simulink model "c00002M_harness"  (R2018a)
settings: Solver=FixedStepAuto  StartTime=0.0  StopTime=300  FixedStep=0.1  RelTol=1e-3
undefined symbols (not defined in the file): A1, hmax, R1, R2, sigbuilder_block, TempThreshold
(part 4 of 14)

== system c00002M_harness/M221 ==
  note: VALUES
      | ---------------------------------
      | ControlType = 1 | 2 | 3
      | FillTank = 0 | 1
      | EmptyTank = 0 | 1
      | ManualReference between 0 and 1
      | Tempreature between 0 and 100
      | EmergencyButton = 0 | 1
      | LiquidLevel between 0 and 1 (hmax)
  note: Inputs For Tank2
  note: NAMES
      | --------------------------------------------
      | CT1 = ControlType Tank 1
      | F1 = Fill Tank 1
      | E1 = Empty Tank 1
      | MR1 = Manual Reference Tank1
      | T1 = Temperature Tank 1
      | EB1 = Emergency Button Tank 1
      | LL1 = Liquid Level 1
  note: Inputs For Tank3
  note: Inputs For Tank1
  CT1 : Inport
  MR1 : Inport  Port=2
  T1 : Inport  Port=3
  EB1 : Inport  Port=4
  CT3 : Inport  Port=5
  MR3 : Inport  Port=6
  T3 : Inport  Port=7
  EB3 : Inport  Port=8
  Tank1 : Subsystem
  Tank3 : Subsystem
  LL1 : Outport
  LL3 : Outport  Port=2
  wires:
  EB1/1 -> Tank1/4(EB1)
  Tank3/1(LL3) -> LL3/1
  MR3/1 -> Tank3/2(MR3)
  MR1/1 -> Tank1/2(MR1)
  T1/1 -> Tank1/3(T1)
  Tank1/1(LL1) -> LL1/1
  CT3/1 -> Tank3/1(CT3)
  EB3/1 -> Tank3/4(EB3)
  T3/1 -> Tank3/3(T3)
  CT1/1 -> Tank1/1(CT1)

== system c00002M_harness/M222 ==
  note: VALUES
      | ---------------------------------
      | ControlType = 1 | 2 | 3
      | FillTank = 0 | 1
      | EmptyTank = 0 | 1
      | ManualReference between 0 and 1
      | Tempreature between 0 and 100
      | EmergencyButton = 0 | 1
      | LiquidLevel between 0 and 1 (hmax)
  note: Inputs For Tank2
  note: NAMES
      | --------------------------------------------
      | CT1 = ControlType Tank 1
      | F1 = Fill Tank 1
      | E1 = Empty Tank 1
      | MR1 = Manual Reference Tank1
      | T1 = Temperature Tank 1
      | EB1 = Emergency Button Tank 1
      | LL1 = Liquid Level 1
  note: Inputs For Tank3
  note: Inputs For Tank1
  CT1 : Inport
  MR1 : Inport  Port=2
  T1 : Inport  Port=3
  EB1 : Inport  Port=4
  CT3 : Inport  Port=5
  MR3 : Inport  Port=6
  T3 : Inport  Port=7
  EB3 : Inport  Port=8
  Tank1 : Subsystem
  Tank3 : Subsystem
  LL1 : Outport
  LL3 : Outport  Port=2
  wires:
  EB1/1 -> Tank1/4(EB1)
  Tank3/1(LL3) -> LL3/1
  MR3/1 -> Tank3/2(MR3)
  MR1/1 -> Tank1/2(MR1)
  T1/1 -> Tank1/3(T1)
  Tank1/1(LL1) -> LL1/1
  CT3/1 -> Tank3/1(CT3)
  EB3/1 -> Tank3/4(EB3)
  T3/1 -> Tank3/3(T3)
  CT1/1 -> Tank1/1(CT1)

== system c00002M_harness/M223 ==
  note: VALUES
      | ---------------------------------
      | ControlType = 1 | 2 | 3
      | FillTank = 0 | 1
      | EmptyTank = 0 | 1
      | ManualReference between 0 and 1
      | Tempreature between 0 and 100
      | EmergencyButton = 0 | 1
      | LiquidLevel between 0 and 1 (hmax)
  note: Inputs For Tank2
  note: NAMES
      | --------------------------------------------
      | CT1 = ControlType Tank 1
      | F1 = Fill Tank 1
      | E1 = Empty Tank 1
      | MR1 = Manual Reference Tank1
      | T1 = Temperature Tank 1
      | EB1 = Emergency Button Tank 1
      | LL1 = Liquid Level 1
  note: Inputs For Tank3
  note: Inputs For Tank1
  CT1 : Inport
  MR1 : Inport  Port=2
  T1 : Inport  Port=3
  EB1 : Inport  Port=4
  CT3 : Inport  Port=5
  MR3 : Inport  Port=6
  T3 : Inport  Port=7
  EB3 : Inport  Port=8
  Tank1 : Subsystem
  Tank3 : Subsystem
  LL1 : Outport
  LL3 : Outport  Port=2
  wires:
  EB1/1 -> Tank1/4(EB1)
  Tank3/1(LL3) -> LL3/1
  MR3/1 -> Tank3/2(MR3)
  MR1/1 -> Tank1/2(MR1)
  T1/1 -> Tank1/3(T1)
  Tank1/1(LL1) -> LL1/1
  CT3/1 -> Tank3/1(CT3)
  EB3/1 -> Tank3/4(EB3)
  T3/1 -> Tank3/3(T3)
  CT1/1 -> Tank1/1(CT1)

== system c00002M_harness/M224 ==
  note: VALUES
      | ---------------------------------
      | ControlType = 1 | 2 | 3
      | FillTank = 0 | 1
      | EmptyTank = 0 | 1
      | ManualReference between 0 and 1
      | Tempreature between 0 and 100
      | EmergencyButton = 0 | 1
      | LiquidLevel between 0 and 1 (hmax)
  note: Inputs For Tank2
  note: NAMES
      | --------------------------------------------
      | CT1 = ControlType Tank 1
      | F1 = Fill Tank 1
      | E1 = Empty Tank 1
      | MR1 = Manual Reference Tank1
      | T1 = Temperature Tank 1
      | EB1 = Emergency Button Tank 1
      | LL1 = Liquid Level 1
  note: Inputs For Tank3
  note: Inputs For Tank1
  CT1 : Inport
  MR1 : Inport  Port=2
  T1 : Inport  Port=3
  EB1 : Inport  Port=4
  CT3 : Inport  Port=5
  MR3 : Inport  Port=6
  T3 : Inport  Port=7
  EB3 : Inport  Port=8
  Tank1 : Subsystem
  Tank3 : Subsystem
  LL1 : Outport
  LL3 : Outport  Port=2
  wires:
  EB1/1 -> Tank1/4(EB1)
  Tank3/1(LL3) -> LL3/1
  MR3/1 -> Tank3/2(MR3)
  MR1/1 -> Tank1/2(MR1)
  T1/1 -> Tank1/3(T1)
  Tank1/1(LL1) -> LL1/1
  CT3/1 -> Tank3/1(CT3)
  EB3/1 -> Tank3/4(EB3)
  T3/1 -> Tank3/3(T3)
  CT1/1 -> Tank1/1(CT1)

== system c00002M_harness/M225 ==
  note: VALUES
      | ---------------------------------
      | ControlType = 1 | 2 | 3
      | FillTank = 0 | 1
      | EmptyTank = 0 | 1
      | ManualReference between 0 and 1
      | Tempreature between 0 and 100
      | EmergencyButton = 0 | 1
      | LiquidLevel between 0 and 1 (hmax)
  note: Inputs For Tank2
  note: NAMES
      | --------------------------------------------
      | CT1 = ControlType Tank 1
      | F1 = Fill Tank 1
      | E1 = Empty Tank 1
      | MR1 = Manual Reference Tank1
      | T1 = Temperature Tank 1
      | EB1 = Emergency Button Tank 1
      | LL1 = Liquid Level 1
  note: Inputs For Tank3
  note: Inputs For Tank1
  CT1 : Inport
  MR1 : Inport  Port=2
  T1 : Inport  Port=3
  EB1 : Inport  Port=4
  CT3 : Inport  Port=5
  MR3 : Inport  Port=6
  T3 : Inport  Port=7
  EB3 : Inport  Port=8
  Tank1 : Subsystem
  Tank3 : Subsystem
  LL1 : Outport
  LL3 : Outport  Port=2
  wires:
  EB1/1 -> Tank1/4(EB1)
  Tank3/1(LL3) -> LL3/1
  MR3/1 -> Tank3/2(MR3)
  MR1/1 -> Tank1/2(MR1)
  T1/1 -> Tank1/3(T1)
  Tank1/1(LL1) -> LL1/1
  CT3/1 -> Tank3/1(CT3)
  EB3/1 -> Tank3/4(EB3)
  T3/1 -> Tank3/3(T3)
  CT1/1 -> Tank1/1(CT1)

== system c00002M_harness/M233 ==
  note: VALUES
      | ---------------------------------
      | ControlType = 1 | 2 | 3
      | FillTank = 0 | 1
      | EmptyTank = 0 | 1
      | ManualReference between 0 and 1
      | Tempreature between 0 and 100
      | EmergencyButton = 0 | 1
      | LiquidLevel between 0 and 1 (hmax)
  note: Inputs For Tank2
  note: NAMES
      | --------------------------------------------
      | CT1 = ControlType Tank 1
      | F1 = Fill Tank 1
      | E1 = Empty Tank 1
      | MR1 = Manual Reference Tank1
      | T1 = Temperature Tank 1
      | EB1 = Emergency Button Tank 1
      | LL1 = Liquid Level 1
  note: Inputs For Tank3
  note: Inputs For Tank1
  CT1 : Inport
  MR1 : Inport  Port=2
  T1 : Inport  Port=3
  EB1 : Inport  Port=4
  CT3 : Inport  Port=5
  MR3 : Inport  Port=6
  T3 : Inport  Port=7
  EB3 : Inport  Port=8
  Tank1 : Subsystem
  Tank3 : Subsystem
  LL1 : Outport
  LL3 : Outport  Port=2
  wires:
  EB1/1 -> Tank1/4(EB1)
  Tank3/1(LL3) -> LL3/1
  MR3/1 -> Tank3/2(MR3)
  MR1/1 -> Tank1/2(MR1)
  T1/1 -> Tank1/3(T1)
  Tank1/1(LL1) -> LL1/1
  CT3/1 -> Tank3/1(CT3)
  EB3/1 -> Tank3/4(EB3)
  T3/1 -> Tank3/3(T3)
  CT1/1 -> Tank1/1(CT1)

== system c00002M_harness/M234 ==
  note: VALUES
      | ---------------------------------
      | ControlType = 1 | 2 | 3
      | FillTank = 0 | 1
      | EmptyTank = 0 | 1
      | ManualReference between 0 and 1
      | Tempreature between 0 and 100
      | EmergencyButton = 0 | 1
      | LiquidLevel between 0 and 1 (hmax)
  note: Inputs For Tank2
  note: NAMES
      | --------------------------------------------
      | CT1 = ControlType Tank 1
      | F1 = Fill Tank 1
      | E1 = Empty Tank 1
      | MR1 = Manual Reference Tank1
      | T1 = Temperature Tank 1
      | EB1 = Emergency Button Tank 1
      | LL1 = Liquid Level 1
  note: Inputs For Tank3
  note: Inputs For Tank1
  CT1 : Inport
  MR1 : Inport  Port=2
  T1 : Inport  Port=3
  EB1 : Inport  Port=4
  CT3 : Inport  Port=5
  MR3 : Inport  Port=6
  T3 : Inport  Port=7
  EB3 : Inport  Port=8
  Tank1 : Subsystem
  Tank3 : Subsystem
  LL1 : Outport
  LL3 : Outport  Port=2
  wires:
  EB1/1 -> Tank1/4(EB1)
  Tank3/1(LL3) -> LL3/1
  MR3/1 -> Tank3/2(MR3)
  MR1/1 -> Tank1/2(MR1)
  T1/1 -> Tank1/3(T1)
  Tank1/1(LL1) -> LL1/1
  CT3/1 -> Tank3/1(CT3)
  EB3/1 -> Tank3/4(EB3)
  T3/1 -> Tank3/3(T3)
  CT1/1 -> Tank1/1(CT1)

== system c00002M_harness/M235 ==
  note: VALUES
      | ---------------------------------
      | ControlType = 1 | 2 | 3
      | FillTank = 0 | 1
      | EmptyTank = 0 | 1
      | ManualReference between 0 and 1
      | Tempreature between 0 and 100
      | EmergencyButton = 0 | 1
      | LiquidLevel between 0 and 1 (hmax)
  note: Inputs For Tank2
  note: NAMES
      | --------------------------------------------
      | CT1 = ControlType Tank 1
      | F1 = Fill Tank 1
      | E1 = Empty Tank 1
      | MR1 = Manual Reference Tank1
      | T1 = Temperature Tank 1
      | EB1 = Emergency Button Tank 1
      | LL1 = Liquid Level 1
  note: Inputs For Tank3
  note: Inputs For Tank1
  CT1 : Inport
  MR1 : Inport  Port=2
  T1 : Inport  Port=3
  EB1 : Inport  Port=4
  CT3 : Inport  Port=5
  MR3 : Inport  Port=6
  T3 : Inport  Port=7
  EB3 : Inport  Port=8
  Tank1 : Subsystem
  Tank3 : Subsystem
  LL1 : Outport
  LL3 : Outport  Port=2
  wires:
  EB1/1 -> Tank1/4(EB1)
  Tank3/1(LL3) -> LL3/1
  MR3/1 -> Tank3/2(MR3)
  MR1/1 -> Tank1/2(MR1)
  T1/1 -> Tank1/3(T1)
  Tank1/1(LL1) -> LL1/1
  CT3/1 -> Tank3/1(CT3)
  EB3/1 -> Tank3/4(EB3)
  T3/1 -> Tank3/3(T3)
  CT1/1 -> Tank1/1(CT1)

== system c00002M_harness/M236 ==
  note: VALUES
      | ---------------------------------
      | ControlType = 1 | 2 | 3
      | FillTank = 0 | 1
      | EmptyTank = 0 | 1
      | ManualReference between 0 and 1
      | Tempreature between 0 and 100
      | EmergencyButton = 0 | 1
      | LiquidLevel between 0 and 1 (hmax)
  note: Inputs For Tank2
  note: NAMES
      | --------------------------------------------
      | CT1 = ControlType Tank 1
      | F1 = Fill Tank 1
      | E1 = Empty Tank 1
      | MR1 = Manual Reference Tank1
      | T1 = Temperature Tank 1
      | EB1 = Emergency Button Tank 1
      | LL1 = Liquid Level 1
  note: Inputs For Tank3
  note: Inputs For Tank1
  CT1 : Inport
  MR1 : Inport  Port=2
  T1 : Inport  Port=3
  EB1 : Inport  Port=4
  CT3 : Inport  Port=5
  MR3 : Inport  Port=6
  T3 : Inport  Port=7
  EB3 : Inport  Port=8
  Tank1 : Subsystem
  Tank3 : Subsystem
  LL1 : Outport
  LL3 : Outport  Port=2
  wires:
  EB1/1 -> Tank1/4(EB1)
  Tank3/1(LL3) -> LL3/1
  MR3/1 -> Tank3/2(MR3)
  MR1/1 -> Tank1/2(MR1)
  T1/1 -> Tank1/3(T1)
  Tank1/1(LL1) -> LL1/1
  CT3/1 -> Tank3/1(CT3)
  EB3/1 -> Tank3/4(EB3)
  T3/1 -> Tank3/3(T3)
  CT1/1 -> Tank1/1(CT1)

== system c00002M_harness/M237 ==
  note: VALUES
      | ---------------------------------
      | ControlType = 1 | 2 | 3
      | FillTank = 0 | 1
      | EmptyTank = 0 | 1
      | ManualReference between 0 and 1
      | Tempreature between 0 and 100
      | EmergencyButton = 0 | 1
      | LiquidLevel between 0 and 1 (hmax)
  note: Inputs For Tank2
  note: NAMES
      | --------------------------------------------
      | CT1 = ControlType Tank 1
      | F1 = Fill Tank 1
      | E1 = Empty Tank 1
      | MR1 = Manual Reference Tank1
      | T1 = Temperature Tank 1
      | EB1 = Emergency Button Tank 1
      | LL1 = Liquid Level 1
  note: Inputs For Tank3
  note: Inputs For Tank1
  CT1 : Inport
  MR1 : Inport  Port=2
  T1 : Inport  Port=3
  EB1 : Inport  Port=4
  CT3 : Inport  Port=5
  MR3 : Inport  Port=6
  T3 : Inport  Port=7
  EB3 : Inport  Port=8
  Tank1 : Subsystem
  Tank3 : Subsystem
  LL1 : Outport
  LL3 : Outport  Port=2
  wires:
  EB1/1 -> Tank1/4(EB1)
  Tank3/1(LL3) -> LL3/1
  MR3/1 -> Tank3/2(MR3)
  MR1/1 -> Tank1/2(MR1)
  T1/1 -> Tank1/3(T1)
  Tank1/1(LL1) -> LL1/1
  CT3/1 -> Tank3/1(CT3)
  EB3/1 -> Tank3/4(EB3)
  T3/1 -> Tank3/3(T3)
  CT1/1 -> Tank1/1(CT1)

== system c00002M_harness/M238 ==
  note: VALUES
      | ---------------------------------
      | ControlType = 1 | 2 | 3
      | FillTank = 0 | 1
      | EmptyTank = 0 | 1
      | ManualReference between 0 and 1
      | Tempreature between 0 and 100
      | EmergencyButton = 0 | 1
      | LiquidLevel between 0 and 1 (hmax)
  note: Inputs For Tank2
  note: NAMES
      | --------------------------------------------
      | CT1 = ControlType Tank 1
      | F1 = Fill Tank 1
      | E1 = Empty Tank 1
      | MR1 = Manual Reference Tank1
      | T1 = Temperature Tank 1
      | EB1 = Emergency Button Tank 1
      | LL1 = Liquid Level 1
  note: Inputs For Tank3
  note: Inputs For Tank1
  CT1 : Inport
  MR1 : Inport  Port=2
  T1 : Inport  Port=3
  EB1 : Inport  Port=4
  CT3 : Inport  Port=5
  MR3 : Inport  Port=6
  T3 : Inport  Port=7
  EB3 : Inport  Port=8
  Tank1 : Subsystem
  Tank3 : Subsystem
  LL1 : Outport
  LL3 : Outport  Port=2
  wires:
  EB1/1 -> Tank1/4(EB1)
  Tank3/1(LL3) -> LL3/1
  MR3/1 -> Tank3/2(MR3)
  MR1/1 -> Tank1/2(MR1)
  T1/1 -> Tank1/3(T1)
  Tank1/1(LL1) -> LL1/1
  CT3/1 -> Tank3/1(CT3)
  EB3/1 -> Tank3/4(EB3)
  T3/1 -> Tank3/3(T3)
  CT1/1 -> Tank1/1(CT1)

== system c00002M_harness/M239 ==
  note: VALUES
      | ---------------------------------
      | ControlType = 1 | 2 | 3
      | FillTank = 0 | 1
      | EmptyTank = 0 | 1
      | ManualReference between 0 and 1
      | Tempreature between 0 and 100
      | EmergencyButton = 0 | 1
      | LiquidLevel between 0 and 1 (hmax)
  note: Inputs For Tank2
  note: NAMES
      | --------------------------------------------
      | CT1 = ControlType Tank 1
      | F1 = Fill Tank 1
      | E1 = Empty Tank 1
      | MR1 = Manual Reference Tank1
      | T1 = Temperature Tank 1
      | EB1 = Emergency Button Tank 1
      | LL1 = Liquid Level 1
  note: Inputs For Tank3
  note: Inputs For Tank1
  CT1 : Inport
  MR1 : Inport  Port=2
  T1 : Inport  Port=3
  EB1 : Inport  Port=4
  CT3 : Inport  Port=5
  MR3 : Inport  Port=6
  T3 : Inport  Port=7
  EB3 : Inport  Port=8
  Tank1 : Subsystem
  Tank3 : Subsystem
  LL1 : Outport
  LL3 : Outport  Port=2
  wires:
  EB1/1 -> Tank1/4(EB1)
  Tank3/1(LL3) -> LL3/1
  MR3/1 -> Tank3/2(MR3)
  MR1/1 -> Tank1/2(MR1)
  T1/1 -> Tank1/3(T1)
  Tank1/1(LL1) -> LL1/1
  CT3/1 -> Tank3/1(CT3)
  EB3/1 -> Tank3/4(EB3)
  T3/1 -> Tank3/3(T3)
  CT1/1 -> Tank1/1(CT1)

== system c00002M_harness/M240 ==
  note: VALUES
      | ---------------------------------
      | ControlType = 1 | 2 | 3
      | FillTank = 0 | 1
      | EmptyTank = 0 | 1
      | ManualReference between 0 and 1
      | Tempreature between 0 and 100
      | EmergencyButton = 0 | 1
      | LiquidLevel between 0 and 1 (hmax)
  note: Inputs For Tank2
  note: NAMES
      | --------------------------------------------
      | CT1 = ControlType Tank 1
      | F1 = Fill Tank 1
      | E1 = Empty Tank 1
      | MR1 = Manual Reference Tank1
      | T1 = Temperature Tank 1
      | EB1 = Emergency Button Tank 1
      | LL1 = Liquid Level 1
  note: Inputs For Tank3
  note: Inputs For Tank1
  CT1 : Inport
  MR1 : Inport  Port=2
  T1 : Inport  Port=3
  EB1 : Inport  Port=4
  CT3 : Inport  Port=5
  MR3 : Inport  Port=6
  T3 : Inport  Port=7
  EB3 : Inport  Port=8
  Tank1 : Subsystem
  Tank3 : Subsystem
  LL1 : Outport
  LL3 : Outport  Port=2
  wires:
  EB1/1 -> Tank1/4(EB1)
  Tank3/1(LL3) -> LL3/1
  MR3/1 -> Tank3/2(MR3)
  MR1/1 -> Tank1/2(MR1)
  T1/1 -> Tank1/3(T1)
  Tank1/1(LL1) -> LL1/1
  CT3/1 -> Tank3/1(CT3)
  EB3/1 -> Tank3/4(EB3)
  T3/1 -> Tank3/3(T3)
  CT1/1 -> Tank1/1(CT1)

== system c00002M_harness/M241 ==
  note: VALUES
      | ---------------------------------
      | ControlType = 1 | 2 | 3
      | FillTank = 0 | 1
      | EmptyTank = 0 | 1
      | ManualReference between 0 and 1
      | Tempreature between 0 and 100
      | EmergencyButton = 0 | 1
      | LiquidLevel between 0 and 1 (hmax)
  note: Inputs For Tank2
  note: NAMES
      | --------------------------------------------
      | CT1 = ControlType Tank 1
      | F1 = Fill Tank 1
      | E1 = Empty Tank 1
      | MR1 = Manual Reference Tank1
      | T1 = Temperature Tank 1
      | EB1 = Emergency Button Tank 1
      | LL1 = Liquid Level 1
  note: Inputs For Tank3
  note: Inputs For Tank1
  CT1 : Inport
  MR1 : Inport  Port=2
  T1 : Inport  Port=3
  EB1 : Inport  Port=4
  CT3 : Inport  Port=5
  MR3 : Inport  Port=6
  T3 : Inport  Port=7
  EB3 : Inport  Port=8
  Tank1 : Subsystem
  Tank3 : Subsystem
  LL1 : Outport
  LL3 : Outport  Port=2
  wires:
  EB1/1 -> Tank1/4(EB1)
  Tank3/1(LL3) -> LL3/1
  MR3/1 -> Tank3/2(MR3)
  MR1/1 -> Tank1/2(MR1)
  T1/1 -> Tank1/3(T1)
  Tank1/1(LL1) -> LL1/1
  CT3/1 -> Tank3/1(CT3)
  EB3/1 -> Tank3/4(EB3)
  T3/1 -> Tank3/3(T3)
  CT1/1 -> Tank1/1(CT1)

== system c00002M_harness/M242 ==
  note: VALUES
      | ---------------------------------
      | ControlType = 1 | 2 | 3
      | FillTank = 0 | 1
      | EmptyTank = 0 | 1
      | ManualReference between 0 and 1
      | Tempreature between 0 and 100
      | EmergencyButton = 0 | 1
      | LiquidLevel between 0 and 1 (hmax)
  note: Inputs For Tank2
  note: NAMES
      | --------------------------------------------
      | CT1 = ControlType Tank 1
      | F1 = Fill Tank 1
      | E1 = Empty Tank 1
      | MR1 = Manual Reference Tank1
      | T1 = Temperature Tank 1
      | EB1 = Emergency Button Tank 1
      | LL1 = Liquid Level 1
  note: Inputs For Tank3
  note: Inputs For Tank1
  CT1 : Inport
  MR1 : Inport  Port=2
  T1 : Inport  Port=3
  EB1 : Inport  Port=4
  CT3 : Inport  Port=5
  MR3 : Inport  Port=6
  T3 : Inport  Port=7
  EB3 : Inport  Port=8
  Tank1 : Subsystem
  Tank3 : Subsystem
  LL1 : Outport
  LL3 : Outport  Port=2
  wires:
  EB1/1 -> Tank1/4(EB1)
  Tank3/1(LL3) -> LL3/1
  MR3/1 -> Tank3/2(MR3)
  MR1/1 -> Tank1/2(MR1)
  T1/1 -> Tank1/3(T1)
  Tank1/1(LL1) -> LL1/1
  CT3/1 -> Tank3/1(CT3)
  EB3/1 -> Tank3/4(EB3)
  T3/1 -> Tank3/3(T3)
  CT1/1 -> Tank1/1(CT1)

== system c00002M_harness/M243 ==
  note: VALUES
      | ---------------------------------
      | ControlType = 1 | 2 | 3
      | FillTank = 0 | 1
      | EmptyTank = 0 | 1
      | ManualReference between 0 and 1
      | Tempreature between 0 and 100
      | EmergencyButton = 0 | 1
      | LiquidLevel between 0 and 1 (hmax)
  note: Inputs For Tank2
  note: NAMES
      | --------------------------------------------
      | CT1 = ControlType Tank 1
      | F1 = Fill Tank 1
      | E1 = Empty Tank 1
      | MR1 = Manual Reference Tank1
      | T1 = Temperature Tank 1
      | EB1 = Emergency Button Tank 1
      | LL1 = Liquid Level 1
  note: Inputs For Tank3
  note: Inputs For Tank1
  CT1 : Inport
  MR1 : Inport  Port=2
  T1 : Inport  Port=3
  EB1 : Inport  Port=4
  CT3 : Inport  Port=5
  MR3 : Inport  Port=6
  T3 : Inport  Port=7
  EB3 : Inport  Port=8
  Tank1 : Subsystem
  Tank3 : Subsystem
  LL1 : Outport
  LL3 : Outport  Port=2
  wires:
  EB1/1 -> Tank1/4(EB1)
  Tank3/1(LL3) -> LL3/1
  MR3/1 -> Tank3/2(MR3)
  MR1/1 -> Tank1/2(MR1)
  T1/1 -> Tank1/3(T1)
  Tank1/1(LL1) -> LL1/1
  CT3/1 -> Tank3/1(CT3)
  EB3/1 -> Tank3/4(EB3)
  T3/1 -> Tank3/3(T3)
  CT1/1 -> Tank1/1(CT1)

== system c00002M_harness/M244 ==
  note: VALUES
      | ---------------------------------
      | ControlType = 1 | 2 | 3
      | FillTank = 0 | 1
      | EmptyTank = 0 | 1
      | ManualReference between 0 and 1
      | Tempreature between 0 and 100
      | EmergencyButton = 0 | 1
      | LiquidLevel between 0 and 1 (hmax)
  note: Inputs For Tank2
  note: NAMES
      | --------------------------------------------
      | CT1 = ControlType Tank 1
      | F1 = Fill Tank 1
      | E1 = Empty Tank 1
      | MR1 = Manual Reference Tank1
      | T1 = Temperature Tank 1
      | EB1 = Emergency Button Tank 1
      | LL1 = Liquid Level 1
  note: Inputs For Tank3
  note: Inputs For Tank1
  CT1 : Inport
  MR1 : Inport  Port=2
  T1 : Inport  Port=3
  EB1 : Inport  Port=4
  CT3 : Inport  Port=5
  MR3 : Inport  Port=6
  T3 : Inport  Port=7
  EB3 : Inport  Port=8
  Tank1 : Subsystem
  Tank3 : Subsystem
  LL1 : Outport
  LL3 : Outport  Port=2
  wires:
  EB1/1 -> Tank1/4(EB1)
  Tank3/1(LL3) -> LL3/1
  MR3/1 -> Tank3/2(MR3)
  MR1/1 -> Tank1/2(MR1)
  T1/1 -> Tank1/3(T1)
  Tank1/1(LL1) -> LL1/1
  CT3/1 -> Tank3/1(CT3)
  EB3/1 -> Tank3/4(EB3)
  T3/1 -> Tank3/3(T3)
  CT1/1 -> Tank1/1(CT1)

== system c00002M_harness/M245 ==
  note: VALUES
      | ---------------------------------
      | ControlType = 1 | 2 | 3
      | FillTank = 0 | 1
      | EmptyTank = 0 | 1
      | ManualReference between 0 and 1
      | Tempreature between 0 and 100
      | EmergencyButton = 0 | 1
      | LiquidLevel between 0 and 1 (hmax)
  note: Inputs For Tank2
  note: NAMES
      | --------------------------------------------
      | CT1 = ControlType Tank 1
      | F1 = Fill Tank 1
      | E1 = Empty Tank 1
      | MR1 = Manual Reference Tank1
      | T1 = Temperature Tank 1
      | EB1 = Emergency Button Tank 1
      | LL1 = Liquid Level 1
  note: Inputs For Tank3
  note: Inputs For Tank1
  CT1 : Inport
  MR1 : Inport  Port=2
  T1 : Inport  Port=3
  EB1 : Inport  Port=4
  CT3 : Inport  Port=5
  MR3 : Inport  Port=6
  T3 : Inport  Port=7
  EB3 : Inport  Port=8
  Tank1 : Subsystem
  Tank3 : Subsystem
  LL1 : Outport
  LL3 : Outport  Port=2
  wires:
  EB1/1 -> Tank1/4(EB1)
  Tank3/1(LL3) -> LL3/1
  MR3/1 -> Tank3/2(MR3)
  MR1/1 -> Tank1/2(MR1)
  T1/1 -> Tank1/3(T1)
  Tank1/1(LL1) -> LL1/1
  CT3/1 -> Tank3/1(CT3)
  EB3/1 -> Tank3/4(EB3)
  T3/1 -> Tank3/3(T3)
  CT1/1 -> Tank1/1(CT1)

== system c00002M_harness/M246 ==
  note: VALUES
      | ---------------------------------
      | ControlType = 1 | 2 | 3
      | FillTank = 0 | 1
      | EmptyTank = 0 | 1
      | ManualReference between 0 and 1
      | Tempreature between 0 and 100
      | EmergencyButton = 0 | 1
      | LiquidLevel between 0 and 1 (hmax)
  note: Inputs For Tank2
  note: NAMES
      | --------------------------------------------
      | CT1 = ControlType Tank 1
      | F1 = Fill Tank 1
      | E1 = Empty Tank 1
      | MR1 = Manual Reference Tank1
      | T1 = Temperature Tank 1
      | EB1 = Emergency Button Tank 1
      | LL1 = Liquid Level 1
  note: Inputs For Tank3
  note: Inputs For Tank1
  CT1 : Inport
  MR1 : Inport  Port=2
  T1 : Inport  Port=3
  EB1 : Inport  Port=4
  CT3 : Inport  Port=5
  MR3 : Inport  Port=6
  T3 : Inport  Port=7
  EB3 : Inport  Port=8
  Tank1 : Subsystem
  Tank3 : Subsystem
  LL1 : Outport
  LL3 : Outport  Port=2
  wires:
  EB1/1 -> Tank1/4(EB1)
  Tank3/1(LL3) -> LL3/1
  MR3/1 -> Tank3/2(MR3)
  MR1/1 -> Tank1/2(MR1)
  T1/1 -> Tank1/3(T1)
  Tank1/1(LL1) -> LL1/1
  CT3/1 -> Tank3/1(CT3)
  EB3/1 -> Tank3/4(EB3)
  T3/1 -> Tank3/3(T3)
  CT1/1 -> Tank1/1(CT1)

== system c00002M_harness/CPSUT/Tank1 ==
  CT1 : Inport
  MR1 : Inport  Port=2
  T1 : Inport  Port=3
  EB1 : Inport  Port=4
  Control : Subsystem
  Memory : Memory
  TankModel : Subsystem
  LL1 : Outport
  wires:
  TankModel/1(LiquidLevel) -> Memory/1, LL1/1
  Control/2(LiquidOut) -> TankModel/2(LiquidOut)
  Memory/1 -> Control/5(LiquidLevel)
  MR1/1 -> Control/2(ManualReference)
  CT1/1 -> Control/1(ControlType)
  EB1/1 -> Control/3(EmergencyButton)
  T1/1 -> Control/4(Temperature)
  Control/1(LiquidIn) -> TankModel/1(LiquidIn)

== system c00002M_harness/CPSUT/Tank3 ==
  CT3 : Inport
  MR3 : Inport  Port=2
  T3 : Inport  Port=3
  EB3 : Inport  Port=4
  Control : Subsystem
  Memory : Memory
  TankModel : Subsystem
  LL3 : Outport
  wires:
  TankModel/1(LiquidLevel) -> Memory/1, LL3/1
  Control/2(LiquidOut) -> TankModel/2(LiquidOut)
  Memory/1 -> Control/5(LiquidLevel)
  MR3/1 -> Control/2(ManualReference)
  CT3/1 -> Control/1(ControlType)
  EB3/1 -> Control/3(EmergencyButton)
  T3/1 -> Control/4(Temperature)
  Control/1(LiquidIn) -> TankModel/1(LiquidIn)

== system c00002M_harness/M001/Tank1 ==
  CT1 : Inport
  MR1 : Inport  Port=2
  T1 : Inport  Port=3
  EB1 : Inport  Port=4
  Control : Subsystem
  Memory : Memory
  TankModel : Subsystem
  LL1 : Outport
  wires:
  T1/1 -> Control/4(Temperature)
  EB1/1 -> Control/3(EmergencyButton)
  CT1/1 -> Control/1(ControlType)
  MR1/1 -> Control/2(ManualReference)
  Memory/1 -> Control/5(LiquidLevel)
  Control/2(LiquidOut) -> TankModel/2(LiquidOut)
  TankModel/1(LiquidLevel) -> LL1/1, Memory/1
  Control/1(LiquidIn) -> TankModel/1(LiquidIn)

== system c00002M_harness/M001/Tank3 ==
  CT3 : Inport
  MR3 : Inport  Port=2
  T3 : Inport  Port=3
  EB3 : Inport  Port=4
  Control : Subsystem
  Memory : Memory
  TankModel : Subsystem
  LL3 : Outport
  wires:
  T3/1 -> Control/4(Temperature)
  EB3/1 -> Control/3(EmergencyButton)
  CT3/1 -> Control/1(ControlType)
  MR3/1 -> Control/2(ManualReference)
  Memory/1 -> Control/5(LiquidLevel)
  Control/2(LiquidOut) -> TankModel/2(LiquidOut)
  TankModel/1(LiquidLevel) -> LL3/1, Memory/1
  Control/1(LiquidIn) -> TankModel/1(LiquidIn)

== system c00002M_harness/M002/Tank1 ==
  CT1 : Inport
  MR1 : Inport  Port=2
  T1 : Inport  Port=3
  EB1 : Inport  Port=4
  Control : Subsystem
  Memory : Memory
  TankModel : Subsystem
  LL1 : Outport
  wires:
  TankModel/1(LiquidLevel) -> Memory/1, LL1/1
  Control/2(LiquidOut) -> TankModel/2(LiquidOut)
  Memory/1 -> Control/5(LiquidLevel)
  MR1/1 -> Control/2(ManualReference)
  CT1/1 -> Control/1(ControlType)
  EB1/1 -> Control/3(EmergencyButton)
  T1/1 -> Control/4(Temperature)
  Control/1(LiquidIn) -> TankModel/1(LiquidIn)

== system c00002M_harness/M002/Tank3 ==
  CT3 : Inport
  MR3 : Inport  Port=2
  T3 : Inport  Port=3
  EB3 : Inport  Port=4
  Control : Subsystem
  Memory : Memory
  TankModel : Subsystem
  LL3 : Outport
  wires:
  TankModel/1(LiquidLevel) -> Memory/1, LL3/1
  Control/2(LiquidOut) -> TankModel/2(LiquidOut)
  Memory/1 -> Control/5(LiquidLevel)
  MR3/1 -> Control/2(ManualReference)
  CT3/1 -> Control/1(ControlType)
  EB3/1 -> Control/3(EmergencyButton)
  T3/1 -> Control/4(Temperature)
  Control/1(LiquidIn) -> TankModel/1(LiquidIn)

== system c00002M_harness/M003/Tank1 ==
  CT1 : Inport
  MR1 : Inport  Port=2
  T1 : Inport  Port=3
  EB1 : Inport  Port=4
  Control : Subsystem
  Memory : Memory
  TankModel : Subsystem
  LL1 : Outport
  wires:
  TankModel/1(LiquidLevel) -> Memory/1, LL1/1
  Control/2(LiquidOut) -> TankModel/2(LiquidOut)
  Memory/1 -> Control/5(LiquidLevel)
  MR1/1 -> Control/2(ManualReference)
  CT1/1 -> Control/1(ControlType)
  EB1/1 -> Control/3(EmergencyButton)
  T1/1 -> Control/4(Temperature)
  Control/1(LiquidIn) -> TankModel/1(LiquidIn)

== system c00002M_harness/M003/Tank3 ==
  CT3 : Inport
  MR3 : Inport  Port=2
  T3 : Inport  Port=3
  EB3 : Inport  Port=4
  Control : Subsystem
  Memory : Memory
  TankModel : Subsystem
  LL3 : Outport
  wires:
  TankModel/1(LiquidLevel) -> Memory/1, LL3/1
  Control/2(LiquidOut) -> TankModel/2(LiquidOut)
  Memory/1 -> Control/5(LiquidLevel)
  MR3/1 -> Control/2(ManualReference)
  CT3/1 -> Control/1(ControlType)
  EB3/1 -> Control/3(EmergencyButton)
  T3/1 -> Control/4(Temperature)
  Control/1(LiquidIn) -> TankModel/1(LiquidIn)

== system c00002M_harness/M004/Tank1 ==
  CT1 : Inport
  MR1 : Inport  Port=2
  T1 : Inport  Port=3
  EB1 : Inport  Port=4
  Control : Subsystem
  Memory : Memory
  TankModel : Subsystem
  LL1 : Outport
  wires:
  TankModel/1(LiquidLevel) -> Memory/1, LL1/1
  Control/2(LiquidOut) -> TankModel/2(LiquidOut)
  Memory/1 -> Control/5(LiquidLevel)
  MR1/1 -> Control/2(ManualReference)
  CT1/1 -> Control/1(ControlType)
  EB1/1 -> Control/3(EmergencyButton)
  T1/1 -> Control/4(Temperature)
  Control/1(LiquidIn) -> TankModel/1(LiquidIn)

== system c00002M_harness/M004/Tank3 ==
  CT3 : Inport
  MR3 : Inport  Port=2
  T3 : Inport  Port=3
  EB3 : Inport  Port=4
  Control : Subsystem
  Memory : Memory
  TankModel : Subsystem
  LL3 : Outport
  wires:
  TankModel/1(LiquidLevel) -> Memory/1, LL3/1
  Control/2(LiquidOut) -> TankModel/2(LiquidOut)
  Memory/1 -> Control/5(LiquidLevel)
  MR3/1 -> Control/2(ManualReference)
  CT3/1 -> Control/1(ControlType)
  EB3/1 -> Control/3(EmergencyButton)
  T3/1 -> Control/4(Temperature)
  Control/1(LiquidIn) -> TankModel/1(LiquidIn)

== system c00002M_harness/M046/Tank1 ==
  CT1 : Inport
  MR1 : Inport  Port=2
  T1 : Inport  Port=3
  EB1 : Inport  Port=4
  Control : Subsystem
  Memory : Memory
  TankModel : Subsystem
  LL1 : Outport
  wires:
  TankModel/1(LiquidLevel) -> Memory/1, LL1/1
  Control/2(LiquidOut) -> TankModel/2(LiquidOut)
  Memory/1 -> Control/5(LiquidLevel)
  MR1/1 -> Control/2(ManualReference)
  CT1/1 -> Control/1(ControlType)
  EB1/1 -> Control/3(EmergencyButton)
  T1/1 -> Control/4(Temperature)
  Control/1(LiquidIn) -> TankModel/1(LiquidIn)

== system c00002M_harness/M046/Tank3 ==
  CT3 : Inport
  MR3 : Inport  Port=2
  T3 : Inport  Port=3
  EB3 : Inport  Port=4
  Control : Subsystem
  Memory : Memory
  TankModel : Subsystem
  LL3 : Outport
  wires:
  TankModel/1(LiquidLevel) -> Memory/1, LL3/1
  Control/2(LiquidOut) -> TankModel/2(LiquidOut)
  Memory/1 -> Control/5(LiquidLevel)
  MR3/1 -> Control/2(ManualReference)
  CT3/1 -> Control/1(ControlType)
  EB3/1 -> Control/3(EmergencyButton)
  T3/1 -> Control/4(Temperature)
  Control/1(LiquidIn) -> TankModel/1(LiquidIn)

== system c00002M_harness/M047/Tank1 ==
  CT1 : Inport
  MR1 : Inport  Port=2
  T1 : Inport  Port=3
  EB1 : Inport  Port=4
  Control : Subsystem
  Memory : Memory
  TankModel : Subsystem
  LL1 : Outport
  wires:
  TankModel/1(LiquidLevel) -> Memory/1, LL1/1
  Control/2(LiquidOut) -> TankModel/2(LiquidOut)
  Memory/1 -> Control/5(LiquidLevel)
  MR1/1 -> Control/2(ManualReference)
  CT1/1 -> Control/1(ControlType)
  EB1/1 -> Control/3(EmergencyButton)
  T1/1 -> Control/4(Temperature)
  Control/1(LiquidIn) -> TankModel/1(LiquidIn)

== system c00002M_harness/M047/Tank3 ==
  CT3 : Inport
  MR3 : Inport  Port=2
  T3 : Inport  Port=3
  EB3 : Inport  Port=4
  Control : Subsystem
  Memory : Memory
  TankModel : Subsystem
  LL3 : Outport
  wires:
  TankModel/1(LiquidLevel) -> Memory/1, LL3/1
  Control/2(LiquidOut) -> TankModel/2(LiquidOut)
  Memory/1 -> Control/5(LiquidLevel)
  MR3/1 -> Control/2(ManualReference)
  CT3/1 -> Control/1(ControlType)
  EB3/1 -> Control/3(EmergencyButton)
  T3/1 -> Control/4(Temperature)
  Control/1(LiquidIn) -> TankModel/1(LiquidIn)

== system c00002M_harness/M048/Tank1 ==
  CT1 : Inport
  MR1 : Inport  Port=2
  T1 : Inport  Port=3
  EB1 : Inport  Port=4
  Control : Subsystem
  Memory : Memory
  TankModel : Subsystem
  LL1 : Outport
  wires:
  TankModel/1(LiquidLevel) -> Memory/1, LL1/1
  Control/2(LiquidOut) -> TankModel/2(LiquidOut)
  Memory/1 -> Control/5(LiquidLevel)
  MR1/1 -> Control/2(ManualReference)
  CT1/1 -> Control/1(ControlType)
  EB1/1 -> Control/3(EmergencyButton)
  T1/1 -> Control/4(Temperature)
  Control/1(LiquidIn) -> TankModel/1(LiquidIn)

== system c00002M_harness/M048/Tank3 ==
  CT3 : Inport
  MR3 : Inport  Port=2
  T3 : Inport  Port=3
  EB3 : Inport  Port=4
  Control : Subsystem
  Memory : Memory
  TankModel : Subsystem
  LL3 : Outport
  wires:
  TankModel/1(LiquidLevel) -> Memory/1, LL3/1
  Control/2(LiquidOut) -> TankModel/2(LiquidOut)
  Memory/1 -> Control/5(LiquidLevel)
  MR3/1 -> Control/2(ManualReference)
  CT3/1 -> Control/1(ControlType)
  EB3/1 -> Control/3(EmergencyButton)
  T3/1 -> Control/4(Temperature)
  Control/1(LiquidIn) -> TankModel/1(LiquidIn)

== system c00002M_harness/M049/Tank1 ==
  CT1 : Inport
  MR1 : Inport  Port=2
  T1 : Inport  Port=3
  EB1 : Inport  Port=4
  Control : Subsystem
  Memory : Memory
  TankModel : Subsystem
  LL1 : Outport
  wires:
  TankModel/1(LiquidLevel) -> Memory/1, LL1/1
  Control/2(LiquidOut) -> TankModel/2(LiquidOut)
  Memory/1 -> Control/5(LiquidLevel)
  MR1/1 -> Control/2(ManualReference)
  CT1/1 -> Control/1(ControlType)
  EB1/1 -> Control/3(EmergencyButton)
  T1/1 -> Control/4(Temperature)
  Control/1(LiquidIn) -> TankModel/1(LiquidIn)

== system c00002M_harness/M049/Tank3 ==
  CT3 : Inport
  MR3 : Inport  Port=2
  T3 : Inport  Port=3
  EB3 : Inport  Port=4
  Control : Subsystem
  Memory : Memory
  TankModel : Subsystem
  LL3 : Outport
  wires:
  TankModel/1(LiquidLevel) -> Memory/1, LL3/1
  Control/2(LiquidOut) -> TankModel/2(LiquidOut)
  Memory/1 -> Control/5(LiquidLevel)
  MR3/1 -> Control/2(ManualReference)
  CT3/1 -> Control/1(ControlType)
  EB3/1 -> Control/3(EmergencyButton)
  T3/1 -> Control/4(Temperature)
  Control/1(LiquidIn) -> TankModel/1(LiquidIn)

== system c00002M_harness/M050/Tank1 ==
  CT1 : Inport
  MR1 : Inport  Port=2
  T1 : Inport  Port=3
  EB1 : Inport  Port=4
  Control : Subsystem
  Memory : Memory
  TankModel : Subsystem
  LL1 : Outport
  wires:
  TankModel/1(LiquidLevel) -> Memory/1, LL1/1
  Control/2(LiquidOut) -> TankModel/2(LiquidOut)
  Memory/1 -> Control/5(LiquidLevel)
  MR1/1 -> Control/2(ManualReference)
  CT1/1 -> Control/1(ControlType)
  EB1/1 -> Control/3(EmergencyButton)
  T1/1 -> Control/4(Temperature)
  Control/1(LiquidIn) -> TankModel/1(LiquidIn)

== system c00002M_harness/M050/Tank3 ==
  CT3 : Inport
  MR3 : Inport  Port=2
  T3 : Inport  Port=3
  EB3 : Inport  Port=4
  Control : Subsystem
  Memory : Memory
  TankModel : Subsystem
  LL3 : Outport
  wires:
  TankModel/1(LiquidLevel) -> Memory/1, LL3/1
  Control/2(LiquidOut) -> TankModel/2(LiquidOut)
  Memory/1 -> Control/5(LiquidLevel)
  MR3/1 -> Control/2(ManualReference)
  CT3/1 -> Control/1(ControlType)
  EB3/1 -> Control/3(EmergencyButton)
  T3/1 -> Control/4(Temperature)
  Control/1(LiquidIn) -> TankModel/1(LiquidIn)

== system c00002M_harness/M051/Tank1 ==
  CT1 : Inport
  MR1 : Inport  Port=2
  T1 : Inport  Port=3
  EB1 : Inport  Port=4
  Control : Subsystem
  Memory : Memory
  TankModel : Subsystem
  LL1 : Outport
  wires:
  TankModel/1(LiquidLevel) -> Memory/1, LL1/1
  Control/2(LiquidOut) -> TankModel/2(LiquidOut)
  Memory/1 -> Control/5(LiquidLevel)
  MR1/1 -> Control/2(ManualReference)
  CT1/1 -> Control/1(ControlType)
  EB1/1 -> Control/3(EmergencyButton)
  T1/1 -> Control/4(Temperature)
  Control/1(LiquidIn) -> TankModel/1(LiquidIn)

== system c00002M_harness/M051/Tank3 ==
  CT3 : Inport
  MR3 : Inport  Port=2
  T3 : Inport  Port=3
  EB3 : Inport  Port=4
  Control : Subsystem
  Memory : Memory
  TankModel : Subsystem
  LL3 : Outport
  wires:
  TankModel/1(LiquidLevel) -> Memory/1, LL3/1
  Control/2(LiquidOut) -> TankModel/2(LiquidOut)
  Memory/1 -> Control/5(LiquidLevel)
  MR3/1 -> Control/2(ManualReference)
  CT3/1 -> Control/1(ControlType)
  EB3/1 -> Control/3(EmergencyButton)
  T3/1 -> Control/4(Temperature)
  Control/1(LiquidIn) -> TankModel/1(LiquidIn)

== system c00002M_harness/M052/Tank1 ==
  CT1 : Inport
  MR1 : Inport  Port=2
  T1 : Inport  Port=3
  EB1 : Inport  Port=4
  Control : Subsystem
  Memory : Memory
  TankModel : Subsystem
  LL1 : Outport
  wires:
  TankModel/1(LiquidLevel) -> Memory/1, LL1/1
  Control/2(LiquidOut) -> TankModel/2(LiquidOut)
  Memory/1 -> Control/5(LiquidLevel)
  MR1/1 -> Control/2(ManualReference)
  CT1/1 -> Control/1(ControlType)
  EB1/1 -> Control/3(EmergencyButton)
  T1/1 -> Control/4(Temperature)
  Control/1(LiquidIn) -> TankModel/1(LiquidIn)

== system c00002M_harness/M052/Tank3 ==
  CT3 : Inport
  MR3 : Inport  Port=2
  T3 : Inport  Port=3
  EB3 : Inport  Port=4
  Control : Subsystem
  Memory : Memory
  TankModel : Subsystem
  LL3 : Outport
  wires:
  TankModel/1(LiquidLevel) -> Memory/1, LL3/1
  Control/2(LiquidOut) -> TankModel/2(LiquidOut)
  Memory/1 -> Control/5(LiquidLevel)
  MR3/1 -> Control/2(ManualReference)
  CT3/1 -> Control/1(ControlType)
  EB3/1 -> Control/3(EmergencyButton)
  T3/1 -> Control/4(Temperature)
  Control/1(LiquidIn) -> TankModel/1(LiquidIn)

== system c00002M_harness/M053/Tank1 ==
  CT1 : Inport
  MR1 : Inport  Port=2
  T1 : Inport  Port=3
  EB1 : Inport  Port=4
  Control : Subsystem
  Memory : Memory
  TankModel : Subsystem
  LL1 : Outport
  wires:
  TankModel/1(LiquidLevel) -> Memory/1, LL1/1
  Control/2(LiquidOut) -> TankModel/2(LiquidOut)
  Memory/1 -> Control/5(LiquidLevel)
  MR1/1 -> Control/2(ManualReference)
  CT1/1 -> Control/1(ControlType)
  EB1/1 -> Control/3(EmergencyButton)
  T1/1 -> Control/4(Temperature)
  Control/1(LiquidIn) -> TankModel/1(LiquidIn)

== system c00002M_harness/M053/Tank3 ==
  CT3 : Inport
  MR3 : Inport  Port=2
  T3 : Inport  Port=3
  EB3 : Inport  Port=4
  Control : Subsystem
  Memory : Memory
  TankModel : Subsystem
  LL3 : Outport
  wires:
  TankModel/1(LiquidLevel) -> Memory/1, LL3/1
  Control/2(LiquidOut) -> TankModel/2(LiquidOut)
  Memory/1 -> Control/5(LiquidLevel)
  MR3/1 -> Control/2(ManualReference)
  CT3/1 -> Control/1(ControlType)
  EB3/1 -> Control/3(EmergencyButton)
  T3/1 -> Control/4(Temperature)
  Control/1(LiquidIn) -> TankModel/1(LiquidIn)

== system c00002M_harness/M054/Tank1 ==
  CT1 : Inport
  MR1 : Inport  Port=2
  T1 : Inport  Port=3
  EB1 : Inport  Port=4
  Control : Subsystem
  Memory : Memory
  TankModel : Subsystem
  LL1 : Outport
  wires:
  TankModel/1(LiquidLevel) -> Memory/1, LL1/1
  Control/2(LiquidOut) -> TankModel/2(LiquidOut)
  Memory/1 -> Control/5(LiquidLevel)
  MR1/1 -> Control/2(ManualReference)
  CT1/1 -> Control/1(ControlType)
  EB1/1 -> Control/3(EmergencyButton)
  T1/1 -> Control/4(Temperature)
  Control/1(LiquidIn) -> TankModel/1(LiquidIn)

== system c00002M_harness/M054/Tank3 ==
  CT3 : Inport
  MR3 : Inport  Port=2
  T3 : Inport  Port=3
  EB3 : Inport  Port=4
  Control : Subsystem
  Memory : Memory
  TankModel : Subsystem
  LL3 : Outport
  wires:
  TankModel/1(LiquidLevel) -> Memory/1, LL3/1
  Control/2(LiquidOut) -> TankModel/2(LiquidOut)
  Memory/1 -> Control/5(LiquidLevel)
  MR3/1 -> Control/2(ManualReference)
  CT3/1 -> Control/1(ControlType)
  EB3/1 -> Control/3(EmergencyButton)
  T3/1 -> Control/4(Temperature)
  Control/1(LiquidIn) -> TankModel/1(LiquidIn)

== system c00002M_harness/M055/Tank1 ==
  CT1 : Inport
  MR1 : Inport  Port=2
  T1 : Inport  Port=3
  EB1 : Inport  Port=4
  Control : Subsystem
  Memory : Memory
  TankModel : Subsystem
  LL1 : Outport
  wires:
  TankModel/1(LiquidLevel) -> Memory/1, LL1/1
  Control/2(LiquidOut) -> TankModel/2(LiquidOut)
  Memory/1 -> Control/5(LiquidLevel)
  MR1/1 -> Control/2(ManualReference)
  CT1/1 -> Control/1(ControlType)
  EB1/1 -> Control/3(EmergencyButton)
  T1/1 -> Control/4(Temperature)
  Control/1(LiquidIn) -> TankModel/1(LiquidIn)

== system c00002M_harness/M055/Tank3 ==
  CT3 : Inport
  MR3 : Inport  Port=2
  T3 : Inport  Port=3
  EB3 : Inport  Port=4
  Control : Subsystem
  Memory : Memory
  TankModel : Subsystem
  LL3 : Outport
  wires:
  TankModel/1(LiquidLevel) -> Memory/1, LL3/1
  Control/2(LiquidOut) -> TankModel/2(LiquidOut)
  Memory/1 -> Control/5(LiquidLevel)
  MR3/1 -> Control/2(ManualReference)
  CT3/1 -> Control/1(ControlType)
  EB3/1 -> Control/3(EmergencyButton)
  T3/1 -> Control/4(Temperature)
  Control/1(LiquidIn) -> TankModel/1(LiquidIn)

== system c00002M_harness/M056/Tank1 ==
  CT1 : Inport
  MR1 : Inport  Port=2
  T1 : Inport  Port=3
  EB1 : Inport  Port=4
  Control : Subsystem
  Memory : Memory
  TankModel : Subsystem
  LL1 : Outport
  wires:
  TankModel/1(LiquidLevel) -> Memory/1, LL1/1
  Control/2(LiquidOut) -> TankModel/2(LiquidOut)
  Memory/1 -> Control/5(LiquidLevel)
  MR1/1 -> Control/2(ManualReference)
  CT1/1 -> Control/1(ControlType)
  EB1/1 -> Control/3(EmergencyButton)
  T1/1 -> Control/4(Temperature)
  Control/1(LiquidIn) -> TankModel/1(LiquidIn)

== system c00002M_harness/M056/Tank3 ==
  CT3 : Inport
  MR3 : Inport  Port=2
  T3 : Inport  Port=3
  EB3 : Inport  Port=4
  Control : Subsystem
  Memory : Memory
  TankModel : Subsystem
  LL3 : Outport
  wires:
  TankModel/1(LiquidLevel) -> Memory/1, LL3/1
  Control/2(LiquidOut) -> TankModel/2(LiquidOut)
  Memory/1 -> Control/5(LiquidLevel)
  MR3/1 -> Control/2(ManualReference)
  CT3/1 -> Control/1(ControlType)
  EB3/1 -> Control/3(EmergencyButton)
  T3/1 -> Control/4(Temperature)
  Control/1(LiquidIn) -> TankModel/1(LiquidIn)

== system c00002M_harness/M057/Tank1 ==
  CT1 : Inport
  MR1 : Inport  Port=2
  T1 : Inport  Port=3
  EB1 : Inport  Port=4
  Control : Subsystem
  Memory : Memory
  TankModel : Subsystem
  LL1 : Outport
  wires:
  TankModel/1(LiquidLevel) -> Memory/1, LL1/1
  Control/2(LiquidOut) -> TankModel/2(LiquidOut)
  Memory/1 -> Control/5(LiquidLevel)
  MR1/1 -> Control/2(ManualReference)
  CT1/1 -> Control/1(ControlType)
  EB1/1 -> Control/3(EmergencyButton)
  T1/1 -> Control/4(Temperature)
  Control/1(LiquidIn) -> TankModel/1(LiquidIn)

== system c00002M_harness/M057/Tank3 ==
  CT3 : Inport
  MR3 : Inport  Port=2
  T3 : Inport  Port=3
  EB3 : Inport  Port=4
  Control : Subsystem
  Memory : Memory
  TankModel : Subsystem
  LL3 : Outport
  wires:
  TankModel/1(LiquidLevel) -> Memory/1, LL3/1
  Control/2(LiquidOut) -> TankModel/2(LiquidOut)
  Memory/1 -> Control/5(LiquidLevel)
  MR3/1 -> Control/2(ManualReference)
  CT3/1 -> Control/1(ControlType)
  EB3/1 -> Control/3(EmergencyButton)
  T3/1 -> Control/4(Temperature)
  Control/1(LiquidIn) -> TankModel/1(LiquidIn)

== system c00002M_harness/M058/Tank1 ==
  CT1 : Inport
  MR1 : Inport  Port=2
  T1 : Inport  Port=3
  EB1 : Inport  Port=4
  Control : Subsystem
  Memory : Memory
  TankModel : Subsystem
  LL1 : Outport
  wires:
  TankModel/1(LiquidLevel) -> Memory/1, LL1/1
  Control/2(LiquidOut) -> TankModel/2(LiquidOut)
  Memory/1 -> Control/5(LiquidLevel)
  MR1/1 -> Control/2(ManualReference)
  CT1/1 -> Control/1(ControlType)
  EB1/1 -> Control/3(EmergencyButton)
  T1/1 -> Control/4(Temperature)
  Control/1(LiquidIn) -> TankModel/1(LiquidIn)

== system c00002M_harness/M058/Tank3 ==
  CT3 : Inport
  MR3 : Inport  Port=2
  T3 : Inport  Port=3
  EB3 : Inport  Port=4
  Control : Subsystem
  Memory : Memory
  TankModel : Subsystem
  LL3 : Outport
  wires:
  TankModel/1(LiquidLevel) -> Memory/1, LL3/1
  Control/2(LiquidOut) -> TankModel/2(LiquidOut)
  Memory/1 -> Control/5(LiquidLevel)
  MR3/1 -> Control/2(ManualReference)
  CT3/1 -> Control/1(ControlType)
  EB3/1 -> Control/3(EmergencyButton)
  T3/1 -> Control/4(Temperature)
  Control/1(LiquidIn) -> TankModel/1(LiquidIn)

== system c00002M_harness/M059/Tank1 ==
  CT1 : Inport
  MR1 : Inport  Port=2
  T1 : Inport  Port=3
  EB1 : Inport  Port=4
  Control : Subsystem
  Memory : Memory
  TankModel : Subsystem
  LL1 : Outport
  wires:
  TankModel/1(LiquidLevel) -> Memory/1, LL1/1
  Control/2(LiquidOut) -> TankModel/2(LiquidOut)
  Memory/1 -> Control/5(LiquidLevel)
  MR1/1 -> Control/2(ManualReference)
  CT1/1 -> Control/1(ControlType)
  EB1/1 -> Control/3(EmergencyButton)
  T1/1 -> Control/4(Temperature)
  Control/1(LiquidIn) -> TankModel/1(LiquidIn)

== system c00002M_harness/M059/Tank3 ==
  CT3 : Inport
  MR3 : Inport  Port=2
  T3 : Inport  Port=3
  EB3 : Inport  Port=4
  Control : Subsystem
  Memory : Memory
  TankModel : Subsystem
  LL3 : Outport
  wires:
  TankModel/1(LiquidLevel) -> Memory/1, LL3/1
  Control/2(LiquidOut) -> TankModel/2(LiquidOut)
  Memory/1 -> Control/5(LiquidLevel)
  MR3/1 -> Control/2(ManualReference)
  CT3/1 -> Control/1(ControlType)
  EB3/1 -> Control/3(EmergencyButton)
  T3/1 -> Control/4(Temperature)
  Control/1(LiquidIn) -> TankModel/1(LiquidIn)

== system c00002M_harness/M060/Tank1 ==
  CT1 : Inport
  MR1 : Inport  Port=2
  T1 : Inport  Port=3
  EB1 : Inport  Port=4
  Control : Subsystem
  Memory : Memory
  TankModel : Subsystem
  LL1 : Outport
  wires:
  TankModel/1(LiquidLevel) -> Memory/1, LL1/1
  Control/2(LiquidOut) -> TankModel/2(LiquidOut)
  Memory/1 -> Control/5(LiquidLevel)
  MR1/1 -> Control/2(ManualReference)
  CT1/1 -> Control/1(ControlType)
  EB1/1 -> Control/3(EmergencyButton)
  T1/1 -> Control/4(Temperature)
  Control/1(LiquidIn) -> TankModel/1(LiquidIn)

== system c00002M_harness/M060/Tank3 ==
  CT3 : Inport
  MR3 : Inport  Port=2
  T3 : Inport  Port=3
  EB3 : Inport  Port=4
  Control : Subsystem
  Memory : Memory
  TankModel : Subsystem
  LL3 : Outport
  wires:
  TankModel/1(LiquidLevel) -> Memory/1, LL3/1
  Control/2(LiquidOut) -> TankModel/2(LiquidOut)
  Memory/1 -> Control/5(LiquidLevel)
  MR3/1 -> Control/2(ManualReference)
  CT3/1 -> Control/1(ControlType)
  EB3/1 -> Control/3(EmergencyButton)
  T3/1 -> Control/4(Temperature)
  Control/1(LiquidIn) -> TankModel/1(LiquidIn)

== system c00002M_harness/M061/Tank1 ==
  CT1 : Inport
  MR1 : Inport  Port=2
  T1 : Inport  Port=3
  EB1 : Inport  Port=4
  Control : Subsystem
  Memory : Memory
  TankModel : Subsystem
  LL1 : Outport
  wires:
  TankModel/1(LiquidLevel) -> Memory/1, LL1/1
  Control/2(LiquidOut) -> TankModel/2(LiquidOut)
  Memory/1 -> Control/5(LiquidLevel)
  MR1/1 -> Control/2(ManualReference)
  CT1/1 -> Control/1(ControlType)
  EB1/1 -> Control/3(EmergencyButton)
  T1/1 -> Control/4(Temperature)
  Control/1(LiquidIn) -> TankModel/1(LiquidIn)

== system c00002M_harness/M061/Tank3 ==
  CT3 : Inport
  MR3 : Inport  Port=2
  T3 : Inport  Port=3
  EB3 : Inport  Port=4
  Control : Subsystem
  Memory : Memory
  TankModel : Subsystem
  LL3 : Outport
  wires:
  TankModel/1(LiquidLevel) -> Memory/1, LL3/1
  Control/2(LiquidOut) -> TankModel/2(LiquidOut)
  Memory/1 -> Control/5(LiquidLevel)
  MR3/1 -> Control/2(ManualReference)
  CT3/1 -> Control/1(ControlType)
  EB3/1 -> Control/3(EmergencyButton)
  T3/1 -> Control/4(Temperature)
  Control/1(LiquidIn) -> TankModel/1(LiquidIn)

== system c00002M_harness/M069/Tank1 ==
  CT1 : Inport
  MR1 : Inport  Port=2
  T1 : Inport  Port=3
  EB1 : Inport  Port=4
  Control : Subsystem
  Memory : Memory
  TankModel : Subsystem
  LL1 : Outport
  wires:
  TankModel/1(LiquidLevel) -> Memory/1, LL1/1
  Control/2(LiquidOut) -> TankModel/2(LiquidOut)
  Memory/1 -> Control/5(LiquidLevel)
  MR1/1 -> Control/2(ManualReference)
  CT1/1 -> Control/1(ControlType)
  EB1/1 -> Control/3(EmergencyButton)
  T1/1 -> Control/4(Temperature)
  Control/1(LiquidIn) -> TankModel/1(LiquidIn)

== system c00002M_harness/M069/Tank3 ==
  CT3 : Inport
  MR3 : Inport  Port=2
  T3 : Inport  Port=3
  EB3 : Inport  Port=4
  Control : Subsystem
  Memory : Memory
  TankModel : Subsystem
  LL3 : Outport
  wires:
  TankModel/1(LiquidLevel) -> Memory/1, LL3/1
  Control/2(LiquidOut) -> TankModel/2(LiquidOut)
  Memory/1 -> Control/5(LiquidLevel)
  MR3/1 -> Control/2(ManualReference)
  CT3/1 -> Control/1(ControlType)
  EB3/1 -> Control/3(EmergencyButton)
  T3/1 -> Control/4(Temperature)
  Control/1(LiquidIn) -> TankModel/1(LiquidIn)

== system c00002M_harness/M070/Tank1 ==
  CT1 : Inport
  MR1 : Inport  Port=2
  T1 : Inport  Port=3
  EB1 : Inport  Port=4
  Control : Subsystem
  Memory : Memory
  TankModel : Subsystem
  LL1 : Outport
  wires:
  TankModel/1(LiquidLevel) -> Memory/1, LL1/1
  Control/2(LiquidOut) -> TankModel/2(LiquidOut)
  Memory/1 -> Control/5(LiquidLevel)
  MR1/1 -> Control/2(ManualReference)
  CT1/1 -> Control/1(ControlType)
  EB1/1 -> Control/3(EmergencyButton)
  T1/1 -> Control/4(Temperature)
  Control/1(LiquidIn) -> TankModel/1(LiquidIn)

== system c00002M_harness/M070/Tank3 ==
  CT3 : Inport
  MR3 : Inport  Port=2
  T3 : Inport  Port=3
  EB3 : Inport  Port=4
  Control : Subsystem
  Memory : Memory
  TankModel : Subsystem
  LL3 : Outport
  wires:
  TankModel/1(LiquidLevel) -> Memory/1, LL3/1
  Control/2(LiquidOut) -> TankModel/2(LiquidOut)
  Memory/1 -> Control/5(LiquidLevel)
  MR3/1 -> Control/2(ManualReference)
  CT3/1 -> Control/1(ControlType)
  EB3/1 -> Control/3(EmergencyButton)
  T3/1 -> Control/4(Temperature)
  Control/1(LiquidIn) -> TankModel/1(LiquidIn)

== system c00002M_harness/M071/Tank1 ==
  CT1 : Inport
  MR1 : Inport  Port=2
  T1 : Inport  Port=3
  EB1 : Inport  Port=4
  Control : Subsystem
  Memory : Memory
  TankModel : Subsystem
  LL1 : Outport
  wires:
  TankModel/1(LiquidLevel) -> Memory/1, LL1/1
  Control/2(LiquidOut) -> TankModel/2(LiquidOut)
  Memory/1 -> Control/5(LiquidLevel)
  MR1/1 -> Control/2(ManualReference)
  CT1/1 -> Control/1(ControlType)
  EB1/1 -> Control/3(EmergencyButton)
  T1/1 -> Control/4(Temperature)
  Control/1(LiquidIn) -> TankModel/1(LiquidIn)

== system c00002M_harness/M071/Tank3 ==
  CT3 : Inport
  MR3 : Inport  Port=2
  T3 : Inport  Port=3
  EB3 : Inport  Port=4
  Control : Subsystem
  Memory : Memory
  TankModel : Subsystem
  LL3 : Outport
  wires:
  TankModel/1(LiquidLevel) -> Memory/1, LL3/1
  Control/2(LiquidOut) -> TankModel/2(LiquidOut)
  Memory/1 -> Control/5(LiquidLevel)
  MR3/1 -> Control/2(ManualReference)
  CT3/1 -> Control/1(ControlType)
  EB3/1 -> Control/3(EmergencyButton)
  T3/1 -> Control/4(Temperature)
  Control/1(LiquidIn) -> TankModel/1(LiquidIn)

== system c00002M_harness/M072/Tank1 ==
  CT1 : Inport
  MR1 : Inport  Port=2
  T1 : Inport  Port=3
  EB1 : Inport  Port=4
  Control : Subsystem
  Memory : Memory
  TankModel : Subsystem
  LL1 : Outport
  wires:
  TankModel/1(LiquidLevel) -> Memory/1, LL1/1
  Control/2(LiquidOut) -> TankModel/2(LiquidOut)
  Memory/1 -> Control/5(LiquidLevel)
  MR1/1 -> Control/2(ManualReference)
  CT1/1 -> Control/1(ControlType)
  EB1/1 -> Control/3(EmergencyButton)
  T1/1 -> Control/4(Temperature)
  Control/1(LiquidIn) -> TankModel/1(LiquidIn)

== system c00002M_harness/M072/Tank3 ==
  CT3 : Inport
  MR3 : Inport  Port=2
  T3 : Inport  Port=3
  EB3 : Inport  Port=4
  Control : Subsystem
  Memory : Memory
  TankModel : Subsystem
  LL3 : Outport
  wires:
  TankModel/1(LiquidLevel) -> Memory/1, LL3/1
  Control/2(LiquidOut) -> TankModel/2(LiquidOut)
  Memory/1 -> Control/5(LiquidLevel)
  MR3/1 -> Control/2(ManualReference)
  CT3/1 -> Control/1(ControlType)
  EB3/1 -> Control/3(EmergencyButton)
  T3/1 -> Control/4(Temperature)
  Control/1(LiquidIn) -> TankModel/1(LiquidIn)

== system c00002M_harness/M073/Tank1 ==
  CT1 : Inport
  MR1 : Inport  Port=2
  T1 : Inport  Port=3
  EB1 : Inport  Port=4
  Control : Subsystem
  Memory : Memory
  TankModel : Subsystem
  LL1 : Outport
  wires:
  TankModel/1(LiquidLevel) -> Memory/1, LL1/1
  Control/2(LiquidOut) -> TankModel/2(LiquidOut)
  Memory/1 -> Control/5(LiquidLevel)
  MR1/1 -> Control/2(ManualReference)
  CT1/1 -> Control/1(ControlType)
  EB1/1 -> Control/3(EmergencyButton)
  T1/1 -> Control/4(Temperature)
  Control/1(LiquidIn) -> TankModel/1(LiquidIn)

== system c00002M_harness/M073/Tank3 ==
  CT3 : Inport
  MR3 : Inport  Port=2
  T3 : Inport  Port=3
  EB3 : Inport  Port=4
  Control : Subsystem
  Memory : Memory
  TankModel : Subsystem
  LL3 : Outport
  wires:
  TankModel/1(LiquidLevel) -> Memory/1, LL3/1
  Control/2(LiquidOut) -> TankModel/2(LiquidOut)
  Memory/1 -> Control/5(LiquidLevel)
  MR3/1 -> Control/2(ManualReference)
  CT3/1 -> Control/1(ControlType)
  EB3/1 -> Control/3(EmergencyButton)
  T3/1 -> Control/4(Temperature)
  Control/1(LiquidIn) -> TankModel/1(LiquidIn)

== system c00002M_harness/M074/Tank1 ==
  CT1 : Inport
  MR1 : Inport  Port=2
  T1 : Inport  Port=3
  EB1 : Inport  Port=4
  Control : Subsystem
  Memory : Memory
  TankModel : Subsystem
  LL1 : Outport
  wires:
  TankModel/1(LiquidLevel) -> Memory/1, LL1/1
  Control/2(LiquidOut) -> TankModel/2(LiquidOut)
  Memory/1 -> Control/5(LiquidLevel)
  MR1/1 -> Control/2(ManualReference)
  CT1/1 -> Control/1(ControlType)
  EB1/1 -> Control/3(EmergencyButton)
  T1/1 -> Control/4(Temperature)
  Control/1(LiquidIn) -> TankModel/1(LiquidIn)

== system c00002M_harness/M074/Tank3 ==
  CT3 : Inport
  MR3 : Inport  Port=2
  T3 : Inport  Port=3
  EB3 : Inport  Port=4
  Control : Subsystem
  Memory : Memory
  TankModel : Subsystem
  LL3 : Outport
  wires:
  TankModel/1(LiquidLevel) -> Memory/1, LL3/1
  Control/2(LiquidOut) -> TankModel/2(LiquidOut)
  Memory/1 -> Control/5(LiquidLevel)
  MR3/1 -> Control/2(ManualReference)
  CT3/1 -> Control/1(ControlType)
  EB3/1 -> Control/3(EmergencyButton)
  T3/1 -> Control/4(Temperature)
  Control/1(LiquidIn) -> TankModel/1(LiquidIn)

== system c00002M_harness/M075/Tank1 ==
  CT1 : Inport
  MR1 : Inport  Port=2
  T1 : Inport  Port=3
  EB1 : Inport  Port=4
  Control : Subsystem
  Memory : Memory
  TankModel : Subsystem
  LL1 : Outport
  wires:
  TankModel/1(LiquidLevel) -> Memory/1, LL1/1
  Control/2(LiquidOut) -> TankModel/2(LiquidOut)
  Memory/1 -> Control/5(LiquidLevel)
  MR1/1 -> Control/2(ManualReference)
  CT1/1 -> Control/1(ControlType)
  EB1/1 -> Control/3(EmergencyButton)
  T1/1 -> Control/4(Temperature)
  Control/1(LiquidIn) -> TankModel/1(LiquidIn)
